simulink model "L03_slide34"  (R2025b)
settings: Solver=FixedStepDiscrete  StartTime=0.0  StopTime=20  FixedStep=0.01*T  RelTol=1e-3  EnableMultiTasking=on
settings Model: Creator=davidecovolo  LastModifiedBy=davidecovolo
settings SolverCC: AlgebraicLoopSolver=TrustRegion  AutoInsertRateTranBlk=on
settings DataIOCC: LimitDataPoints=on
settings OptimizationCC: LifeSpan=inf
settings DebuggingCC: UnconnectedInputMsg=warning  UnconnectedOutputMsg=warning  UnconnectedLineMsg=warning  AllowSymbolicDim=off  SFUnexpectedBacktrackingDiag=warning  SFNoUnconditionalDefaultTransitionDiag=warning  SFExecutionAtInitializationDiag=none  ArithmeticOperatorsInVariantConditions=warning
settings ModelReferenceCC: EnableRefExpFcnMdlSchedulingChecks=on
settings SFSimCC: SimUseLocalCustomCode=off  CustomCodeUndefinedFunction=UseInterfaceOnly
settings RTWCC: RTWUseLocalCustomCode=off  GPUComputeCapability=3.5  DLArmComputeVersion=19.05
settings CodeAppCC: StateflowObjectComments=on
settings GRTTargetCC: TargetLangStandard=C89/C90 (ANSI)
settings ConfigComp: CovMetricSettings=dw  CovSaveCumulativeToWorkspaceVar=on  CovSaveSingleToWorkspaceVar=on  CovExternalEMLEnable=off  CovSFcnEnable=off

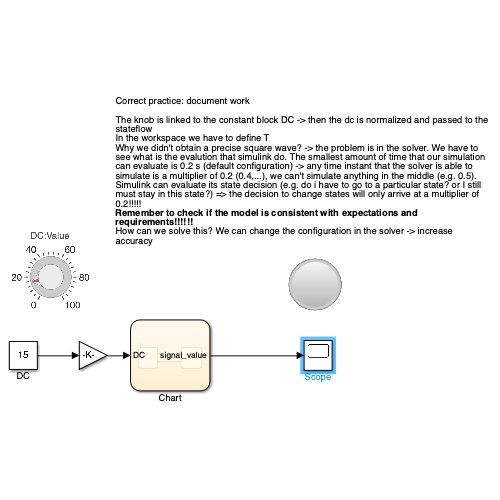
[thumbnail: Simulink's stored preview of the top-level diagram]
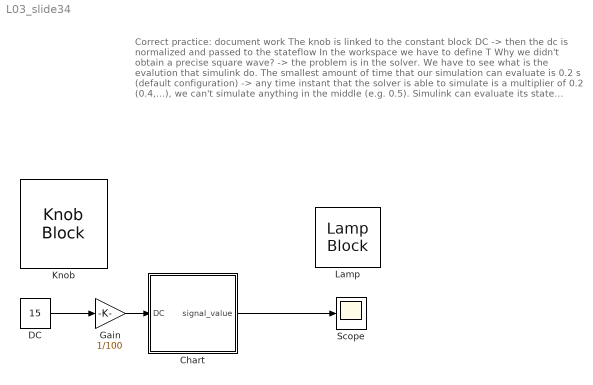
== system L03_slide34 ==
  note: Correct practice: document work
      |
      | The knob is linked to the constant block DC -> then the dc is normalized and passed to the stateflow
      | In the workspace we have to define T
      | Why we didn't obtain a precise square wave? -> the problem is in the solver. We have to see what is the evalution that simulink do. The smallest amount of time that our simulation can evaluate is 0.2 s (default configuration) -> any time instant that the solver is able to simulate is a multiplier of 0.2 (0.4,...), we can't simulate anything in the middle (e.g. 0.5). Simulink can evaluate its state decision (e.g. do i have to go to a particular state? or I still must stay in this state?) => the decision to change states will only arrive at a multiplier of 0.2!!!!!
      | Remember to check if the model is consistent with expectations and requirements!!!!!!
      | How can we solve this? We can change the configuration in the solver -> increase accuracy
  Chart : Stateflow chart  TreatAsAtomicUnit=on
  DC : Constant  Value=15
  Gain : Gain  Gain=1/100
  Knob : KnobBlock
  Lamp : LampBlock  LabelPosition=Hide  DefaultColor=[192.0, 192.0, 192.0]
  Scope : Scope
      settings: ActiveDisplayYMinimum=-0.12499999999999997  ActiveDisplayYMaximum=1.125
  wires:
  Chart/1(signal_value) -> Scope/1
  Gain/1 -> Chart/1(DC)
  DC/1 -> Gain/1

== stateflow chart L03_slide34/Chart ==
  state signal_up
    entry:
    T = T;
    signal_value = 1;
  state signal_down_
    entry:
    signal_value = 0;
  (default) -> signal_up
  signal_up -> signal_down_ : [after(DC*T,sec)]
  signal_down_ -> signal_up : after((1-DC)*T,sec)
  data: DC input; signal_value output; T local =T
